simulink model "NMC_batt_model_100_1dot5C"  (R2023b)
settings: Solver=FixedStepAuto  StartTime=0.0  StopTime=10^7  FixedStep=50
undefined symbols (not defined in the file or in its folder): DiscIntNeverNeededParam, sigbuilder_block
libraries: batteryecm_lib x100, fl_lib x15, nesl_utility x10, simulink x2, dspswit3 x2
(part 1 of 4)
settings Model: Creator=OADEBAJO  LastModifiedBy=OADEBAJO
settings SolverCC: ZeroCrossAlgorithm=Adaptive

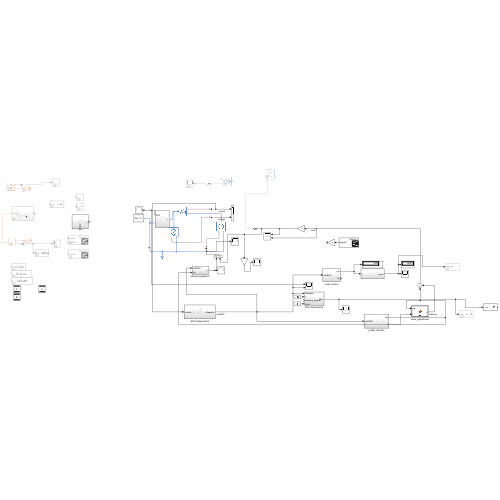
[thumbnail: Simulink's stored preview of the top-level diagram]
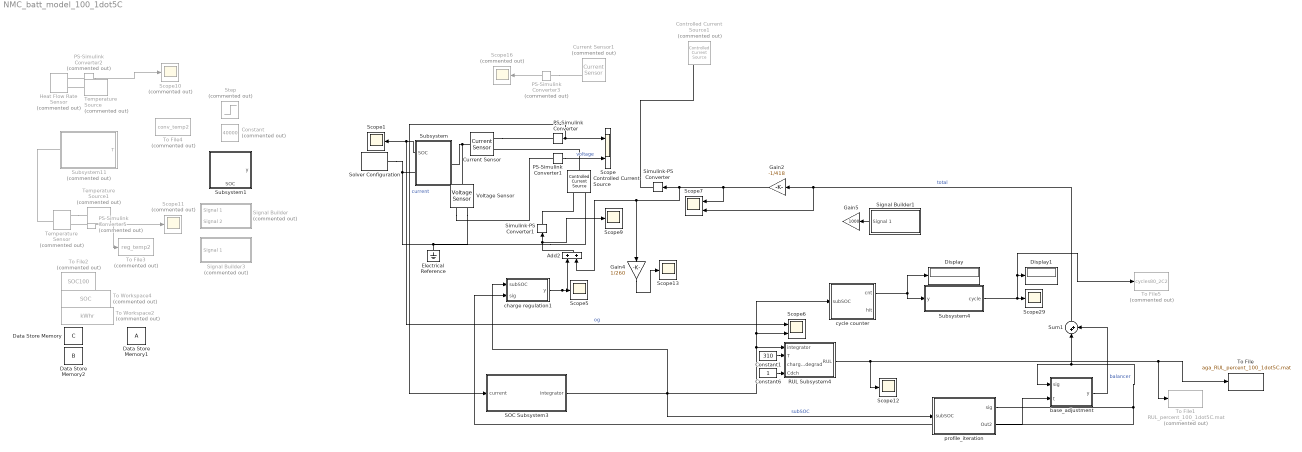
== system NMC_batt_model_100_1dot5C ==
  Add2 : Sum
  Constant : Constant  Commented=on  Value=40000
  Constant1 : Constant  Value=310
  Constant6 : Constant
  Controlled Current Source : fl_lib/Electrical/Electrical Sources/Controlled Current Source
  Controlled Current Source1 : fl_lib/Electrical/Electrical Sources/Controlled Current Source  Commented=on
  Current Sensor : fl_lib/Electrical/Electrical Sensors/Current Sensor
  Current Sensor1 : fl_lib/Electrical/Electrical Sensors/Current Sensor  Commented=on
  Data Store Memory : DataStoreMemory  DataStoreName=C  ReadBeforeWriteMsg=warning  WriteAfterWriteMsg=warning  WriteAfterReadMsg=warning  InitialValue=|  ShowAdditionalParam=off  OutDataTypeStr=double
      | [2000
      | 31300
      | 31300
      | 31300
      | 31300
      | 31300
      | 31300
      | 31300
      | 31300
      | 31300
      | 31300
      | 31300
      | 31300
      | 31300
      | 31300
      | 31300
      | 31300
      | 31300
      | 31300
      | 31300
      | 31300
      | 31300
      | 30655
      | 29990.5
      | 29960.5
      | 32605
      | 35210
      | 34000
      | 30450
      | 30526.67
      | 30460
      | 32000
      | 31716.67
      | 39932.84
      | 39885.07
      | 39837.31
      | 39789.55
      | 39212.64
      | 39210.82
      | 39209
      | 39207.18
      | 39205.36
      | 39203.55
      | 39201.73
      | 39199.91
      | 39198.09
      | 39196.27
      | 39194.45
      | 39192.64
      | 39190.82
      | 39189
      | 39187.18
      | 39185.36
      | 39183.55
      | 39181.73
      | 39179.91
      | 39178.09
      | 39176.27
      | 39174.45
      | 39024.33
      | 38949.38
      | 38948.69
      | 38948
      | 38947.31
      | 38946.62
      | 38945.93
      | 38945.24
      | 38944.55
      | 38943.86
      | 38943.17
      | 38942.48
      | 38941.79
      | 38941.1
      | 38940.41
      | 38939.72
      | 38939.03
      | 38938.34
      | 38937.65
      | 38936.96
      | 38936.27
      | 38935.58
      | 38934.89
      | 38934.2
      | 38933.51
      | 38932.82
      | 38932.13
      | 38931.44
      | 38930.75
      | 38930.06
      | 38929.37
      | 38928.68
      | 38927.99
      | 38927.3
      | 38926.61
      | 38925.92
      | 38925.23
      | 38924.54
      | 38923.85
      | 38923.16
      | 38922.47
      | 38921.79
      | 38921.1
      | 38920.41
      | 38919.72
      | 38919.03
      | 38918.34
      | 38917.65
      | 38916.96
      | 38916.27
      | 38915.58
      | 38914.89
      | 38914.2
      | 38913.51
      | 38912.82
      | 38912.13
      | 38911.44
      | 38910.75
      | 38910.06
      | 38909.37
      | 38908.68
      | 38907.99
      | 38907.3
      | 38906.61
      | 38905.92
      | 38905.23
      | 38904.54
      | 38903.85
      | 38903.16
      | 38902.47
      | 38901.78
      | 38901.09
      | 38900.4
      | 38899.71
      | 38899.02
      | 38898.33
      | 38897.64
      | 38896.95
      | 38896.26
      | 38895.57
      | 38894.88
      | 38894.19
      | 38893.5
      | 38892.81
      | 38892.12
      | 38891.43
      | 38890.74
      | 38890.05
      | 38889.36
      | 38888.67
      | 38887.98
      | 38887.29
      | 38886.6
      | 38885.91
      | 38885.22
      | 38884.53
      | 38883.84
      | 38883.15
      | 38882.46
      | 38881.77
      | 38881.08
      | 38880.39
      | 38879.7
      | 38879.01
      | 38878.32
      | 38877.63
      | 38876.94
      | 38876.25
      | 38875.56
      | 38874.87
      | 38874.19
      | 38873.5
      | 38872.81
      | 38872.12
      | 38871.43
      | 38870.74
      | 38870.05
      | 38869.36
      | 38868.67
      | 38867.98
      | 38867.29
      | 38866.6
      | 38865.91
      | 38865.22
      | 38864.53
      | 38863.84
      | 38863.15
      | 38862.46
      | 38861.77
      | 38861.08
      | 38860.39
      | 38859.7
      | 38859.01
      | 38858.32
      | 38857.63
      | 38856.94
      | 38856.25
      | 38855.56
      | 38854.87
      | 38854.18
      | 38853.49
      | 38852.8
      | 38852.11
      | 38851.42
      | 38850.73
      | 38850.04
      | 38849.35
      | 38848.66
      | 38847.97
      | 38847.28
      | 38846.59
      | 38845.9
      | 38845.21
      | 38844.52
      | 38843.83
      | 38843.14
      | 38842.45
      | 38841.76
      | 38841.07
      | 38840.38
      | 38839.69
      | 38839
      | 38838.31
      | 38837.62
      | 38836.93
      | 38836.24
      | 38835.55
      | 38834.86
      | 38834.17
      | 38833.48
      | 38832.79
      | 38832.1
      | 38831.41
      | 38830.72
      | 38830.03
      | 36768.41
      | 35227.5
      | 34141.5
      | 35942.5
      | 33093.33
      | 29998.33
      | 29290
      | 29290
      | 32756.67
      | 30673.33
      | 30960
      | 30067.5
      | 30017.5
      | 2000]
  Data Store Memory1 : DataStoreMemory  ReadBeforeWriteMsg=warning  WriteAfterWriteMsg=warning  WriteAfterReadMsg=warning  InitialValue=|  ShowAdditionalParam=off  OutDataTypeStr=double
      | [2000
      | 31300
      | 31300
      | 31300
      | 31300
      | 31300
      | 31300
      | 31300
      | 31300
      | 30005.5
      | 32605
      | 30040
      | 30460
      | 37653
      | 39837.31343
      | 39211.72727
      | 39207.18182
      | 39202.63636
      | 39198.09091
      | 39193.54545
      | 39189
      | 39184.45455
      | 39179.90909
      | 39175.36364
      | 38949.37913
      | 38947.6545
      | 38945.92986
      | 38944.20523
      | 38942.4806
      | 38940.75596
      | 38939.03133
      | 38937.3067
      | 38935.58206
      | 38933.85743
      | 38932.1328
      | 38930.40816
      | 38928.68353
      | 38926.9589
      | 38925.23426
      | 38923.50963
      | 38921.785
      | 38920.06036
      | 38918.33573
      | 38916.6111
      | 38914.88646
      | 38913.16183
      | 38911.43719
      | 38909.71256
      | 38907.98793
      | 38906.26329
      | 38904.53866
      | 38902.81403
      | 38901.08939
      | 38899.36476
      | 38897.64013
      | 38895.91549
      | 38894.19086
      | 38892.46623
      | 38890.74159
      | 38889.01696
      | 38887.29233
      | 38885.56769
      | 38883.84306
      | 38882.11842
      | 38880.39379
      | 38878.66916
      | 38876.94452
      | 38875.21989
      | 38873.49526
      | 38871.77062
      | 38870.04599
      | 38868.32136
      | 38866.59672
      | 38864.87209
      | 38863.14746
      | 38861.42282
      | 38859.69819
      | 38857.97356
      | 38856.24892
      | 38854.52429
      | 38852.79966
      | 38851.07502
      | 38849.35039
      | 38847.62575
      | 38845.90112
      | 38844.17649
      | 38842.45185
      | 38840.72722
      | 38839.00259
      | 38837.27795
      | 38835.55332
      | 38833.82869
      | 38832.10405
      | 38830.37942
      | 35227.5
      | 36585
      | 29290
      | 32820
      | 16000
      | 2000]
  Data Store Memory2 : DataStoreMemory  DataStoreName=B  WriteAfterWriteMsg=warning  InitialValue=|  ShowAdditionalParam=off  OutDataTypeStr=double
      | [2000
      | 15000
      | 30000
      | 30004.2016806723
      | 30008.4033613445
      | 30012.6050420168
      | 30016.8067226891
      | 30021.0084033613
      | 30025.2100840336
      | 30029.4117647059
      | 30033.6134453782
      | 30037.8151260504
      | 30042.0168067227
      | 30046.2184873950
      | 30050.4201680672
      | 30054.6218487395
      | 30058.8235294118
      | 30063.0252100840
      | 30067.2268907563
      | 30071.4285714286
      | 30075.6302521008
      | 30079.8319327731
      | 30084.0336134454
      | 30088.2352941176
      | 30092.4369747899
      | 30096.6386554622
      | 30100.8403361345
      | 30105.0420168067
      | 30109.2436974790
      | 30113.4453781513
      | 30117.6470588235
      | 30121.8487394958
      | 30126.0504201681
      | 30130.2521008403
      | 30134.4537815126
      | 30138.6554621849
      | 30142.8571428571
      | 30147.0588235294
      | 30151.2605042017
      | 30155.4621848739
      | 30159.6638655462
      | 30163.8655462185
      | 30168.0672268908
      | 30172.2689075630
      | 30176.4705882353
      | 30180.6722689076
      | 30184.8739495798
      | 30189.0756302521
      | 30193.2773109244
      | 30197.4789915966
      | 30201.6806722689
      | 30205.8823529412
      | 30210.0840336134
      | 30214.2857142857
      | 30218.4873949580
      | 30222.6890756303
      | 30226.8907563025
      | 30231.0924369748
      | 30235.2941176471
      | 30239.4957983193
      | 30243.6974789916
      | 30247.8991596639
      | 30252.1008403361
      | 30256.3025210084
      | 30260.5042016807
      | 30264.7058823529
      | 30268.9075630252
      | 30273.1092436975
      | 30277.3109243698
      | 30281.5126050420
      | 30285.7142857143
      | 30289.9159663866
      | 30294.1176470588
      | 30298.3193277311
      | 30302.5210084034
      | 30306.7226890756
      | 30310.9243697479
      | 30315.1260504202
      | 30319.3277310924
      | 30323.5294117647
      | 30327.7310924370
      | 30331.9327731092
      | 30336.1344537815
      | 30340.3361344538
      | 30344.5378151261
      | 30348.7394957983
      | 30352.9411764706
      | 30357.1428571429
      | 30361.3445378151
      | 30365.5462184874
      | 30369.7478991597
      | 30373.9495798319
      | 30378.1512605042
      | 30382.3529411765
      | 30386.5546218487
      | 30390.7563025210
      | 30394.9579831933
      | 30399.1596638655
      | 30403.3613445378
      | 30407.5630252101
      | 30411.7647058824
      | 30415.9663865546
      | 30420.1680672269
      | 30424.3697478992
      | 30428.5714285714
      | 30432.7731092437
      | 30436.9747899160
      | 30441.1764705882
      | 30445.3781512605
      | 30449.5798319328
      | 30453.7815126050
      | 30457.9831932773
      | 30462.1848739496
      | 30466.3865546218
      | 30470.5882352941
      | 30474.7899159664
      | 30478.9915966387
      | 30483.1932773109
      | 30487.3949579832
      | 30491.5966386555
      | 30495.7983193277
      | 30500
      | 30504.2016806723
      | 30508.4033613445
      | 30512.6050420168
      | 30516.8067226891
      | 30521.0084033613
      | 30525.2100840336
      | 30529.4117647059
      | 30533.6134453782
      | 30537.8151260504
      | 30542.0168067227
      | 30546.2184873950
      | 30550.4201680672
      | 30554.6218487395
      | 30558.8235294118
      | 30563.0252100840
      | 30567.2268907563
      | 30571.4285714286
      | 30575.6302521008
      | 30579.8319327731
      | 30584.0336134454
      | 30588.2352941176
      | 30592.4369747899
      | 30596.6386554622
      | 30600.8403361345
      | 30605.0420168067
      | 30609.2436974790
      | 30613.4453781513
      | 30617.6470588235
      | 30621.8487394958
      | 30626.0504201681
      | 30630.2521008403
      | 30634.4537815126
      | 30638.6554621849
      | 30642.8571428571
      | 30647.0588235294
      | 30651.2605042017
      | 30655.4621848739
      | 30659.6638655462
      | 30663.8655462185
      | 30668.0672268908
      | 30672.2689075630
      | 30676.4705882353
      | 30680.6722689076
      | 30684.8739495798
      | 30689.0756302521
      | 30693.2773109244
      | 30697.4789915966
      | 30701.6806722689
      | 30705.8823529412
      | 30710.0840336134
      | 30714.2857142857
      | 30718.4873949580
      | 30722.6890756303
      | 30726.8907563025
      | 30731.0924369748
      | 30735.2941176471
      | 30739.4957983193
      | 30743.6974789916
      | 30747.8991596639
      | 30752.1008403361
      | 30756.3025210084
      | 30760.5042016807
      | 30764.7058823529
      | 30768.9075630252
      | 30773.1092436975
      | 30777.3109243698
      | 30781.5126050420
      | 30785.7142857143
      | 30789.9159663866
      | 30794.1176470588
      | 30798.3193277311
      | 30802.5210084034
      | 30806.7226890756
      | 30810.9243697479
      | 30815.1260504202
      | 30819.3277310924
      | 30823.5294117647
      | 30827.7310924370
      | 30831.9327731092
      | 30836.1344537815
      | 30840.3361344538
      | 30844.5378151261
      | 30848.7394957983
      | 30852.9411764706
      | 30857.1428571429
      | 30861.3445378151
      | 30865.5462184874
      | 30869.7478991597
      | 30873.9495798319
      | 30878.1512605042
      | 30882.3529411765
      | 30886.5546218487
      | 30890.7563025210
      | 30894.9579831933
      | 30899.1596638655
      | 30903.3613445378
      | 30907.5630252101
      | 30911.7647058824
      | 30915.9663865546
      | 30920.1680672269
      | 30924.3697478992
      | 30928.5714285714
      | 30932.7731092437
      | 30936.9747899160
      | 30941.1764705882
      | 30945.3781512605
      | 30949.5798319328
      | 30953.7815126050
      | 30957.9831932773
      | 30962.1848739496
      | 30966.3865546218
      | 30970.5882352941
      | 30974.7899159664
      | 30978.9915966387
      | 30983.1932773109
      | 30987.3949579832
      | 30991.5966386555
      | 30995.7983193277
      | 40000
      | 40000
      | 40000
      | 40000
      | 40000
      | 40000
      | 40000
      | 40000
      | 40000
      | 40000
      | 40000
      | 40000
      | 40000
      | 40000
      | 40000
      | 40000
      | 40000
      | 40000
      | 40000
      | 40000
      | 40000
      | 40000
      | 40000
      | 40000
      | 40000
      | 40000
      | 40000
      | 40000
      | 40000
      | 40000
      | 40000
      | 40000
      | 40000
      | 40000
      | 40000
      | 40000
      | 40000
      | 40000
      | 40000
      | 40000
      | 40000
      | 40000
      | 40000
      | 40000
      | 40000
      | 40000
      | 40000
      | 40000
      | 40000
      | 40000
      | 40000
      | 40000
      | 40000
      | 40000
      | 40000
      | 40000
      | 40000
      | 40000
      | 40000
      | 40000
      | 40000
      | 40000
      | 40000
      | 40000
      | 40000
      | 40000
      | 40000
      | 40000
      | 40000
      | 40000
      | 40000
      | 40000
      | 40000
      | 40000
      | 40000
      | 40000
      | 40000
      | 40000
      | 40000
      | 40000
      | 40000
      | 40000
      | 40000
      | 40000
      | 40000
      | 40000
      | 40000
      | 40000
      | 40000
      | 40000
      | 40000
      | 40000
      | 40000
      | 40000
      | 40000
      | 40000
      | 40000
      | 40000
      | 40000
      | 40000
      | 40000
      | 40000
      | 40000
      | 40000
      | 40000
      | 40000
      | 40000
      | 40000
      | 40000
      | 40000
      | 40000
      | 40000
      | 40000
      | 40000
      | 40000
      | 40000
      | 40000
      | 40000
      | 40000
      | 40000
      | 40000
      | 40000
      | 40000
      | 40000
      | 40000
      | 40000
      | 40000
      | 40000
      | 40000
      | 40000
      | 40000
      | 40000
      | 40000
      | 40000
      | 40000
      | 40000
      | 40000
      | 40000
      | 40000
      | 40000
      | 40000
      | 40000
      | 40000
      | 40000
      | 40000
      | 40000
      | 40000
      | 40000
      | 40000
      | 40000
      | 40000
      | 40000
      | 40000
      | 40000
      | 40000
      | 40000
      | 40000
      | 40000
      | 40000
      | 40000
      | 38000
      | 38000
      | 38000
      | 38000
      | 38000
      | 38000
      | 38000
      | 38000
      | 38000
      | 38000
      | 38000
      | 38000
      | 38000
      | 38000
      | 38000
      | 38000
      | 38000
      | 38000
      | 38000
      | 38000
      | 38000
      | 38000
      | 38000
      | 38000
      | 38000
      | 38000
      | 38000
      | 38000
      | 38000
      | 38000
      | 38000
      | 38000
      | 38000
      | 38000
      | 38000
      | 38000
      | 38000
      | 38000
      | 38000
      | 38000
      | 38000
      | 38000
      | 38000
      | 38000
      | 38000
      | 38000
      | 38000
      | 38000
      | 38000
      | 38000
      | 38000
      | 38000
      | 38000
      | 38000
      | 38000
      | 38000
      | 38000
      | 38000
      | 38000
      | 38000
      | 38000
      | 38000
      | 38000
      | 38000
      | 38000
      | 38000
      | 38000
      | 38000
      | 38000
      | 38000
      | 38000
      | 38000
      | 38000
      | 38000
      | 38000
      | 38000
      | 38000
      | 38000
      | 38000
      | 38000
      | 38000
      | 38000
      | 38000
      | 38000
      | 38000
      | 38000
      | 38000
      | 38000
      | 38000
      | 38000
      | 38000
      | 38000
      | 38000
      | 38000
      | 38000
      | 38000
      | 38000
      | 38000
      | 38000
      | 38000
      | 38000
      | 38000
      | 38000
      | 38000
      | 38000
      | 38000
      | 38000
      | 38000
      | 38000
      | 38000
      | 38000
      | 38000
      | 38000
      | 38000
      | 38000
      | 38000
      | 38000
      | 38000
      | 38000
      | 38000
      | 38000
      | 38000
      | 38000
      | 38000
      | 38000
      | 38000
      | 38000
      | 38000
      | 38000
      | 38000
      | 38000
      | 38000
      | 38000
      | 38000
      | 38000
      | 38000
      | 38000
      | 38000
      | 38000
      | 38000
      | 38000
      | 38000
      | 38000
      | 38000
      | 38000
      | 38000
      | 38000
      | 38000
      | 38000
      | 38000
      | 36000
      | 36000
      | 36000
      | 36000
      | 36000
      | 36000
      | 36000
      | 36000
      | 36000
      | 36000
      | 36000
      | 36000
      | 36000
      | 36000
      | 36000
      | 36000
      | 36000
      | 36000
      | 36000
      | 36000
      | 36000
      | 36000
      | 36000
      | 36000
      | 36000
      | 36000
      | 36000
      | 36000
      | 36000
      | 36000
      | 36000
      | 36000
      | 36000
      | 36000
      | 36000
      | 36000
      | 36000
      | 36000
      | 36000
      | 36000
      | 36000
      | 36000
      | 36000
      | 36000
      | 36000
      | 36000
      | 36000
      | 36000
      | 36000
      | 36000
      | 36000
      | 36000
      | 36000
      | 36000
      | 36000
      | 36000
      | 36000
      | 36000
      | 36000
      | 36000
      | 36000
      | 36000
      | 36000
      | 36000
      | 36000
      | 36000
      | 36000
      | 36000
      | 36000
      | 36000
      | 36000
      | 36000
      | 36000
      | 36000
      | 36000
      | 36000
      | 36000
      | 36000
      | 36000
      | 36000
      | 36000
      | 36000
      | 36000
      | 36000
      | 36000
      | 36000
      | 36000
      | 36000
      | 36000
      | 36000
      | 36000
      | 36000
      | 36000
      | 36000
      | 36000
      | 36000
      | 36000
      | 36000
      | 36000
      | 36000
      | 36000
      | 36000
      | 36000
      | 36000
      | 36000
      | 36000
      | 36000
      | 36000
      | 36000
      | 36000
      | 36000
      | 36000
      | 36000
      | 36000
      | 36000
      | 36000
      | 36000
      | 36000
      | 36000
      | 36000
      | 36000
      | 36000
      | 36000
      | 36000
      | 36000
      | 36000
      | 36000
      | 36000
      | 36000
      | 36000
      | 36000
      | 36000
      | 36000
      | 36000
      | 36000
      | 36000
      | 36000
      | 36000
      | 36000
      | 36000
      | 36000
      | 36000
      | 36000
      | 36000
      | 36000
      | 36000
      | 36000
      | 36000
      | 36000
      | 36000
      | 36000
      | 36000
      | 36000
      | 36000
      | 36000
      | 36000
      | 36000
      | 36000
      | 36000
      | 36000
      | 36000
      | 36000
      | 36000
      | 36000
      | 36000
      | 36000
      | 36000
      | 36000
      | 36000
      | 36000
      | 36000
      | 36000
      | 36000
      | 36000
      | 36000
      | 36000
      | 36000
      | 36000
      | 36000
      | 36000
      | 36000
      | 36000
      | 36000
      | 36000
      | 36000
      | 36000
      | 36000
      | 36000
      | 36000
      | 36000
      | 36000
      | 36000
      | 36000
      | 36000
      | 36000
      | 36000
      | 36000
      | 36000
      | 36000
      | 36000
      | 36000
      | 36000
      | 36000
      | 36000
      | 36000
      | 36000
      | 36000
      | 36000
      | 36000
      | 36000
      | 36000
      | 36000
      | 36000
      | 36000
      | 36000
      | 36000
      | 36000
      | 36000
      | 36000
      | 36000
      | 36000
      | 36000
      | 36000
      | 36000
      | 36000
      | 36000
      | 36000
      | 36000
      | 36000
      | 36000
      | 36000
      | 36000
      | 36000
      | 36000
      | 36000
      | 36000
      | 36000
      | 36000
      | 36000
      | 36000
      | 36000
      | 36000
      | 36000
      | 36000
      | 36000
      | 36000
      | 36000
      | 36000
      | 36000
      | 36000
      | 36000
      | 36000
      | 36000
      | 36000
      | 36000
      | 36000
      | 36000
      | 36000
      | 36000
      | 36000
      | 36000
      | 36000
      | 36000
      | 36000
      | 36000
      | 36000
      | 36000
      | 36000
      | 36000
      | 36000
      | 36000
      | 36000
      | 36000
      | 36000
      | 36000
      | 36000
      | 36000
      | 36000
      | 36000
      | 36000
      | 36000
      | 36000
      | 36000
      | 36000
      | 36000
      | 36000
      | 36000
      | 36000
      | 36000
      | 36000
      | 36000
      | 36000
      | 36000
      | 36000
      | 36000
      | 36000
      | 36000
      | 36000
      | 36000
      | 36000
      | 36000
      | 36000
      | 36000
      | 36000
      | 36000
      | 36000
      | 36000
      | 36000
      | 36000
      | 36000
      | 36000
      | 36000
      | 36000
      | 36000
      | 36000
      | 36000
      | 36000
      | 36000
      | 36000
      | 36000
      | 36000
      | 36000
      | 36000
      | 36000
      | 36000
      | 36000
      | 36000
      | 36000
      | 36000
      | 36000
      | 36000
      | 36000
      | 36000
      | 36000
      | 36000
      | 36000
      | 36000
      | 36000
      | 36000
      | 36000
      | 36000
      | 36000
      | 36000
      | 36000
      | 36000
      | 36000
      | 36000
      | 36000
      | 36000
      | 36000
      | 36000
      | 36000
      | 36000
      | 36000
      | 36000
      | 36000
      | 36000
      | 36000
      | 36000
      | 36000
      | 36000
      | 36000
      | 36000
      | 36000
      | 36000
      | 36000
      | 36000
      | 36000
      | 36000
      | 36000
      | 36000
      | 36000
      | 36000
      | 36000
      | 36000
      | 36000
      | 36000
      | 36000
      | 36000
      | 36000
      | 36000
      | 36000
      | 36000
      | 36000
      | 36000
      | 36000
      | 36000
      | 36000
      | 36000
      | 36000
      | 36000
      | 36000
      | 36000
      | 36000
      | 36000
      | 36000
      | 36000
      | 36000
      | 36000
      | 36000
      | 36000
      | 36000
      | 36000
      | 36000
      | 36000
      | 36000
      | 36000
      | 36000
      | 36000
      | 36000
      | 36000
      | 36000
      | 36000
      | 36000
      | 36000
      | 36000
      | 36000
      | 36000
      | 36000
      | 36000
      | 36000
      | 36000
      | 36000
      | 36000
      | 36000
      | 36000
      | 36000
      | 36000
      | 36000
      | 36000
      | 36000
      | 36000
      | 36000
      | 36000
      | 36000
      | 36000
      | 36000
      | 36000
      | 36000
      | 36000
      | 36000
      | 36000
      | 36000
      | 36000
      | 36000
      | 36000
      | 36000
      | 36000
      | 36000
      | 36000
      | 36000
      | 36000
      | 36000
      | 36000
      | 36000
      | 36000
      | 36000
      | 36000
      | 36000
      | 36000
      | 36000
      | 36000
      | 36000
      | 36000
      | 36000
      | 36000
      | 36000
      | 36000
      | 36000
      | 36000
      | 36000
      | 36000
      | 36000
      | 36000
      | 36000
      | 36000
      | 36000
      | 36000
      | 36000
      | 36000
      | 36000
      | 36000
      | 36000
      | 36000
      | 36000
      | 36000
      | 36000
      | 36000
      | 36000
      | 36000
      | 36000
      | 36000
      | 36000
      | 36000
      | 36000
      | 36000
      | 36000
      | 36000
      | 36000
      | 36000
      | 36000
      | 36000
      | 36000
      | 36000
      | 36000
      | 36000
      | 36000
      | 36000
      | 36000
      | 36000
      | 36000
      | 36000
      | 36000
      | 36000
      | 36000
      | 36000
      | 36000
      | 36000
      | 36000
      | 36000
      | 36000
      | 36000
      | 36000
      | 36000
      | 36000
      | 36000
      | 36000
      | 36000
      | 36000
      | 36000
      | 36000
      | 36000
      | 36000
      | 36000
      | 36000
      | 36000
      | 36000
      | 36000
      | 36000
      | 36000
      | 36000
      | 36000
      | 36000
      | 36000
      | 36000
      | 36000
      | 36000
      | 36000
      | 36000
      | 36000
      | 36000
      | 36000
      | 36000
      | 36000
      | 36000
      | 36000
      | 36000
      | 36000
      | 36000
      | 36000
      | 36000
      | 36000
      | 36000
      | 36000
      | 36000
      | 36000
      | 36000
      | 36000
      | 36000
      | 36000
      | 36000
      | 36000
      | 36000
      | 36000
      | 36000
      | 36000
      | 36000
      | 36000
      | 36000
      | 36000
      | 36000
      | 36000
      | 36000
      | 36000
      | 36000
      | 36000
      | 36000
      | 36000
      | 36000
      | 36000
      | 36000
      | 36000
      | 36000
      | 36000
      | 36000
      | 36000
      | 36000
      | 36000
      | 36000
      | 36000
      | 36000
      | 36000
      | 36000
      | 36000
      | 36000
      | 36000
      | 36000
      | 36000
      | 36000
      | 36000
      | 36000
      | 36000
      | 36000
      | 36000
      | 36000
      | 36000
      | 36000
      | 36000
      | 36000
      | 36000
      | 36000
      | 36000
      | 36000
      | 36000
      | 36000
      | 36000
      | 36000
      | 36000
      | 36000
      | 36000
      | 36000
      | 36000
      | 36000
      | 36000
      | 36000
      | 36000
      | 36000
      | 36000
      | 36000
      | 36000
      | 36000
      | 36000
      | 36000
      | 36000
      | 36000
      | 36000
      | 36000
      | 36000
      | 36000
      | 36000
      | 36000
      | 36000
      | 36000
      | 36000
      | 36000
      | 36000
      | 36000
      | 36000
      | 36000
      | 36000
      | 36000
      | 36000
      | 36000
      | 36000
      | 36000
      | 36000
      | 36000
      | 36000
      | 36000
      | 36000
      | 36000
      | 36000
      | 36000
      | 36000
      | 36000
      | 36000
      | 36000
      | 36000
      | 36000
      | 36000
      | 36000
      | 36000
      | 36000
      | 36000
      | 36000
      | 36000
      | 36000
      | 36000
      | 36000
      | 36000
      | 36000
      | 36000
      | 36000
      | 36000
      | 36000
      | 36000
      | 36000
      | 36000
      | 36000
      | 36000
      | 36000
      | 36000
      | 36000
      | 36000
      | 36000
      | 36000
      | 36000
      | 36000
      | 36000
      | 36000
      | 36000
      | 36000
      | 36000
      | 36000
      | 36000
      | 36000
      | 36000
      | 36000
      | 36000
      | 36000
      | 36000
      | 36000
      | 36000
      | 36000
      | 36000
      | 36000
      | 36000
      | 36000
      | 36000
      | 36000
      | 36000
      | 36000
      | 36000
      | 36000
      | 36000
      | 36000
      | 36000
      | 36000
      | 36000
      | 36000
      | 36000
      | 36000
      | 36000
      | 36000
      | 36000
      | 36000
      | 36000
      | 36000
      | 36000
      | 36000
      | 36000
      | 36000
      | 36000
      | 36000
      | 36000
      | 36000
      | 36000
      | 36000
      | 36000
      | 36000
      | 36000
      | 36000
      | 36000
      | 36000
      | 36000
      | 36000
      | 36000
      | 36000
      | 36000
      | 36000
      | 36000
      | 36000
      | 36000
      | 36000
      | 36000
      | 36000
      | 36000
      | 36000
      | 36000
      | 36000
      | 36000
      | 36000
      | 36000
      | 36000
      | 36000
      | 36000
      | 36000
      | 36000
      | 36000
      | 36000
      | 36000
      | 36000
      | 36000
      | 36000
      | 36000
      | 36000
      | 36000
      | 36000
      | 36000
      | 36000
      | 36000
      | 36000
      | 36000
      | 36000
      | 36000
      | 36000
      | 36000
      | 36000
      | 36000
      | 36000
      | 36000
      | 36000
      | 36000
      | 36000
      | 36000
      | 36000
      | 36000
      | 36000
      | 36000
      | 36000
      | 36000
      | 36000
      | 36000
      | 36000
      | 36000
      | 36000
      | 36000
      | 36000
      | 36000
      | 36000
      | 36000
      | 36000
      | 36000
      | 36000
      | 36000
      | 36000
      | 36000
      | 36000
      | 36000
      | 36000
      | 36000
      | 36000
      | 36000
      | 36000
      | 36000
      | 36000
      | 36000
      | 36000
      | 36000
      | 36000
      | 36000
      | 36000
      | 36000
      | 36000
      | 36000
      | 36000
      | 36000
      | 36000
      | 36000
      | 36000
      | 36000
      | 36000
      | 36000
      | 36000
      | 36000
      | 36000
      | 36000
      | 36000
      | 36000
      | 36000
      | 36000
      | 36000
      | 36000
      | 36000
      | 36000
      | 36000
      | 36000
      | 36000
      | 36000
      | 36000
      | 36000
      | 36000
      | 36000
      | 36000
      | 36000
      | 36000
      | 36000
      | 36000
      | 36000
      | 36000
      | 36000
      | 36000
      | 36000
      | 36000
      | 36000
      | 36000
      | 36000
      | 36000
      | 36000
      | 36000
      | 36000
      | 36000
      | 36000
      | 36000
      | 36000
      | 36000
      | 36000
      | 36000
      | 36000
      | 36000
      | 36000
      | 36000
      | 36000
      | 36000
      | 36000
      | 36000
      | 36000
      | 36000
      | 36000
      | 36000
      | 36000
      | 36000
      | 36000
      | 36000
      | 36000
      | 36000
      | 36000
      | 36000
      | 36000
      | 36000
      | 36000
      | 36000
      | 36000
      | 36000
      | 36000
      | 36000
      | 36000
      | 36000
      | 36000
      | 36000
      | 36000
      | 36000
      | 36000
      | 36000
      | 36000
      | 36000
      | 36000
      | 36000
      | 36000
      | 36000
      | 36000
      | 36000
      | 36000
      | 36000
      | 36000
      | 36000
      | 36000
      | 36000
      | 36000
      | 36000
      | 36000
      | 36000
      | 36000
      | 36000
      | 36000
      | 36000
      | 36000
      | 36000
      | 36000
      | 36000
      | 36000
      | 36000
      | 36000
      | 36000
      | 36000
      | 36000
      | 36000
      | 36000
      | 36000
      | 36000
      | 36000
      | 36000
      | 36000
      | 36000
      | 36000
      | 36000
      | 36000
      | 36000
      | 36000
      | 36000
      | 36000
      | 36000
      | 36000
      | 36000
      | 36000
      | 36000
      | 36000
      | 36000
      | 36000
      | 36000
      | 36000
      | 36000
      | 36000
      | 36000
      | 36000
      | 36000
      | 36000
      | 36000
      | 36000
      | 36000
      | 36000
      | 36000
      | 36000
      | 36000
      | 36000
      | 36000
      | 36000
      | 36000
      | 36000
      | 36000
      | 36000
      | 36000
      | 36000
      | 36000
      | 36000
      | 36000
      | 36000
      | 36000
      | 36000
      | 36000
      | 36000
      | 36000
      | 36000
      | 36000
      | 36000
      | 36000
      | 36000
      | 36000
      | 36000
      | 36000
      | 36000
      | 36000
      | 36000
      | 36000
      | 36000
      | 36000
      | 36000
      | 36000
      | 36000
      | 36000
      | 36000
      | 35850.0000000000
      | 35700.0000000000
      | 35550
      | 35400
      | 35250
      | 35100
      | 34950
      | 34800
      | 34650
      | 34500
      | 34350
      | 34200
      | 34050
      | 33900
      | 33750
      | 33600
      | 33450
      | 33300
      | 33150
      | 33000
      | 33000
      | 33000
      | 33000
      | 33000
      | 33000
      | 33000
      | 33000
      | 33000
      | 33000
      | 33000
      | 33000
      | 33000
      | 33000
      | 33000
      | 33000
      | 33000
      | 33000
      | 33000
      | 33000
      | 33000
      | 33000
      | 33000
      | 33000
      | 33000
      | 33000
      | 33000
      | 33000
      | 33000
      | 33000
      | 32000
      | 32000
      | 32000
      | 32000
      | 32000
      | 32000
      | 32000
      | 32000
      | 32000
      | 32000
      | 32000
      | 32000
      | 32000
      | 32000
      | 32000
      | 32000
      | 32000
      | 32000
      | 32000
      | 32000
      | 32000
      | 32000
      | 32000
      | 32000
      | 32000
      | 32000
      | 32000
      | 32000
      | 32000
      | 32000
      | 32000
      | 32000
      | 32000
      | 32000
      | 32000
      | 32000
      | 32000
      | 32000
      | 32000
      | 32000
      | 32000
      | 32000
      | 32000
      | 32000
      | 32000
      | 32000
      | 32000
      | 32000
      | 32000
      | 32000
      | 32000
      | 32000
      | 32000
      | 32000
      | 32000
      | 32000
      | 32000
      | 32000
      | 32000
      | 32000
      | 32000
      | 32000
      | 32000
      | 32000
      | 32000
      | 32000
      | 32000
      | 32000
      | 32000
      | 32000
      | 32000
      | 32000
      | 32000
      | 32000
      | 32000
      | 32000
      | 32000
      | 32000
      | 32000
      | 32000
      | 32000
      | 32000
      | 32000
      | 32000
      | 32000
      | 32000
      | 32000
      | 32000
      | 32000
      | 32000
      | 32000
      | 32000
      | 32000
      | 32000
      | 32000
      | 32000
      | 32000
      | 32000
      | 32000
      | 32000
      | 32000
      | 32000
      | 32000
      | 32000
      | 32000
      | 32000
      | 32000
      | 32000
      | 32000
      | 32000
      | 32000
      | 32000
      | 32000
      | 32000
      | 32000
      | 32000
      | 32000
      | 32000
      | 32000
      | 32000
      | 32000
      | 32000
      | 32000
      | 32000
      | 32000
      | 32000
      | 32000
      | 32000
      | 32000
      | 32000
      | 32000
      | 32000
      | 32000
      | 32000
      | 32000
      | 32000
      | 32000
      | 32000
      | 32000
      | 32000
      | 32000
      | 32000
      | 32000
      | 32000
      | 32000
      | 32000
      | 32000
      | 32000
      | 32000
      | 16000
      | 2000]
  Display : Display
  Display1 : Display
  Electrical Reference : fl_lib/Electrical/Electrical Elements/Electrical Reference
  Gain2 : Gain  Gain=-1/418
  Gain4 : Gain  Gain=1/260
  Gain5 : Gain  Gain=1000
  Heat Flow Rate Sensor : fl_lib/Thermal/Thermal Sensors/Heat Flow Rate Sensor  Commented=on
  PS-Simulink Converter : nesl_utility/PS-Simulink Converter  PhysicalDomain=network_engine_domain  SubClassName=ps_output  LeftPortType=input  RightPortType=output  PseudoPeriodic=off  Frequencies=[]  VectorFormat=inherit  Unit=inherit  AffineConversion=off
  PS-Simulink Converter1 : nesl_utility/PS-Simulink Converter  PhysicalDomain=network_engine_domain  SubClassName=ps_output  LeftPortType=input  RightPortType=output  PseudoPeriodic=off  Frequencies=[]  VectorFormat=inherit  Unit=inherit  AffineConversion=off
  PS-Simulink Converter2 : nesl_utility/PS-Simulink Converter  Commented=on  PhysicalDomain=network_engine_domain  SubClassName=ps_output  LeftPortType=input  RightPortType=output  PseudoPeriodic=off  Frequencies=[]  VectorFormat=inherit  Unit=inherit  AffineConversion=off
  PS-Simulink Converter3 : nesl_utility/PS-Simulink Converter  Commented=on  PhysicalDomain=network_engine_domain  SubClassName=ps_output  LeftPortType=input  RightPortType=output  PseudoPeriodic=off  Frequencies=[]  VectorFormat=inherit  Unit=inherit  AffineConversion=off
  PS-Simulink Converter5 : nesl_utility/PS-Simulink Converter  Commented=on  PhysicalDomain=network_engine_domain  SubClassName=ps_output  LeftPortType=input  RightPortType=output  PseudoPeriodic=off  Frequencies=[]  VectorFormat=inherit  Unit=inherit  AffineConversion=off
  RUL Subsystem4 : Subsystem
  SOC Subsystem3 : Subsystem
  Scope : Scope  NumInputPorts=2
  Scope{1,5,9,12..13,29} (6 alike) : Scope
  Scope10 : Scope  Commented=on
  Scope11 : Scope  Commented=on
  Scope16 : Scope  Commented=on
  Scope6 : Scope  NumInputPorts=2
  Scope7 : Scope  NumInputPorts=2
  Signal Builder : Subsystem  Tag=STV Subsys  Commented=on  LoadFcn=sigbuilder_block('load');  StartFcn=sigbuilder_block('start');  StopFcn=sigbuilder_block('stop');  ClipboardFcn=sigbuilder_block('clipboard');  mask(Sigbuilder block){tuvar=[0:10]}
      mask help: Simulink:masks:SigbuilderBlock_MD
      mask init:
      | if ~strcmp(get_param(bdroot(gcbh),'SimulationStatus'),'stopped') tuvar = sigbuilder_block('maskInit'); end
      settings: CopyFcn=sigbuilder_block('copy');  DeleteFcn=sigbuilder_block('delete');  ModelCloseFcn=sigbuilder_block('modelClose');  PreSaveFcn=sigbuilder_block('preSave');  PauseFcn=sigbuilder_block('pause');  ContinueFcn=sigbuilder_block('continue');  NameChangeFcn=sigbuilder_block('namechange');  OpenFcn=sigbuilder_block('open',[-104.25 -237 1428 771.75 ]);  CloseFcn=sigbuilder_block('close');
      mask Display: plot(0, 0, 100, 100,[2, 2, 32, 32, 2], [68, 8, 8, 68, 68],[32, 2], [38, 38], [32, 19, 2],[53, 60, 44], [32, 17, 17, 2],[16, 16, 31, 31]);txt = getActiveGroup(gcbh);text(2, 100, txt,'verticalAlignment', 'top');
  Signal Builder1 : Subsystem  Tag=STV Subsys  LoadFcn=sigbuilder_block('load');  StartFcn=sigbuilder_block('start');  StopFcn=sigbuilder_block('stop');  ClipboardFcn=sigbuilder_block('clipboard');  mask(Sigbuilder block){tuvar=[0:10]}
      mask help: Simulink:masks:SigbuilderBlock_MD
      mask init:
      | if ~strcmp(get_param(bdroot(gcbh),'SimulationStatus'),'stopped') tuvar = sigbuilder_block('maskInit'); end
      settings: CopyFcn=sigbuilder_block('copy');  DeleteFcn=sigbuilder_block('delete');  ModelCloseFcn=sigbuilder_block('modelClose');  PreSaveFcn=sigbuilder_block('preSave');  PauseFcn=sigbuilder_block('pause');  ContinueFcn=sigbuilder_block('continue');  NameChangeFcn=sigbuilder_block('namechange');  OpenFcn=sigbuilder_block('open',[6 -153 1428 641.25 ]);  CloseFcn=sigbuilder_block('close');
      mask Display: plot(0, 0, 100, 100,[2, 2, 32, 32, 2], [68, 8, 8, 68, 68],[32, 2], [38, 38], [32, 19, 2],[53, 60, 44], [32, 17, 17, 2],[16, 16, 31, 31]);txt = getActiveGroup(gcbh);text(2, 100, txt,'verticalAlignment', 'top');
  Signal Builder3 : Subsystem  Tag=STV Subsys  Commented=on  LoadFcn=sigbuilder_block('load');  StartFcn=sigbuilder_block('start');  StopFcn=sigbuilder_block('stop');  ClipboardFcn=sigbuilder_block('clipboard');  mask(Sigbuilder block){tuvar=[0:10]}
      mask help: Simulink:masks:SigbuilderBlock_MD
      mask init:
      | if ~strcmp(get_param(bdroot(gcbh),'SimulationStatus'),'stopped') tuvar = sigbuilder_block('maskInit'); end
      settings: CopyFcn=sigbuilder_block('copy');  DeleteFcn=sigbuilder_block('delete');  ModelCloseFcn=sigbuilder_block('modelClose');  PreSaveFcn=sigbuilder_block('preSave');  PauseFcn=sigbuilder_block('pause');  ContinueFcn=sigbuilder_block('continue');  NameChangeFcn=sigbuilder_block('namechange');  OpenFcn=sigbuilder_block('open',[6 30 1428 771.75 ]);  CloseFcn=sigbuilder_block('close');
      mask Display: plot(0, 0, 100, 100,[2, 2, 32, 32, 2], [68, 8, 8, 68, 68],[32, 2], [38, 38], [32, 19, 2],[53, 60, 44], [32, 17, 17, 2],[16, 16, 31, 31]);txt = getActiveGroup(gcbh);text(2, 100, txt,'verticalAlignment', 'top');
  Simulink-PS Converter : nesl_utility/Simulink-PS Converter  PhysicalDomain=network_engine_domain  SubClassName=ps_input  LeftPortType=input  RightPortType=output  PseudoPeriodic=off  Frequencies=[]  NoiseDistribution=none  NoiseParameters=[]  Unit=1  AffineConversion=off  FilteringAndDerivatives=provide  SimscapeFilterOrder=1  InputFilterTimeConstant=0.001  UdotUserProvided=0
  Simulink-PS Converter1 : nesl_utility/Simulink-PS Converter  PhysicalDomain=network_engine_domain  SubClassName=ps_input  LeftPortType=input  RightPortType=output  PseudoPeriodic=off  Frequencies=[]  NoiseDistribution=none  NoiseParameters=[]  Unit=1  AffineConversion=off  FilteringAndDerivatives=provide  SimscapeFilterOrder=1  InputFilterTimeConstant=0.001  UdotUserProvided=0
  Solver Configuration : nesl_utility/Solver Configuration  PhysicalDomain=network_engine_domain  SubClassName=solver  LeftPortType=input  RightPortType=generic  Tones=[]  Harmonics=[]  SimulateNoise=off  Profile=off  UseLocalSampling=off  EnableSwitchedLinearOptims=on  FrequencyDomain=off  UseCCode=off  RelTol=0.001  AbsTol=0.001  MinStep=1e-09  ToWorkspace=off  RevertToSquareIcSolve=off  NumHomotopyIterations=100  PhasorMode=off  PhasorModeNumHarmonics=1  ConsistencySolver=NEWTON_XTOL_AFTER_FTOL  IndexReductionMethod=DerivativeReplacement  DoDC=off  ResidualTolerance=1e-09  ConsistencyTolSource=GLOBAL  ConsistencyAbsTol=0.001  ConsistencyRelTol=0.001  ConsistencyTolFactor=1  UseLocalSolver=off  LocalSolverChoice=NE_BACKWARD_EULER_ADVANCER  ResolveIndetEquations=on  FunctionEvalNumThread=1  LocalSolverSampleTime=0.001  DoFixedCost=off  MaxNonlinIter=3  MaxModeIter=2  ComputeImpulses=off  ImpulseIterations=2  LinearAlgebra=auto  LinearAlgebraNumThread=0  EquationFormulation=NE_TIME_EF  DelaysMemoryBudget=1024  AutomaticFiltering=off  FilteringTimeConstant=0.001  PartitionStorageMethod=AS_NEEDED  PartitionMemoryBudget=1024  PartitionMethod=ROBUST  MultibodyUseLocalSolver=off  MultibodyLocalSolverChoice=ODE1  MultibodyLocalSolverSampleTime=0.001
  Step : Step  Commented=on  Time=5000  Before=40000  After=0  SampleTime=0
  Subsystem : Subsystem
  Subsystem1 : Subsystem
      settings: PortSchema="{\"entries\":[{\"content\":{\"sides\":[{\"content\":{},\"type\":\"ConnectorPlacement.EquallySpacedRectSide\",\"uuid\":\"dc57e3e7-2ad3-48c6-bee1-9177bcd0a010\"},{\"content\":{\"connectorIds\":[\"Out1\"],\"side\":\"RIGHT\"},\"type\":\"ConnectorPlacement.EquallySpacedRectSide\",\"uuid\":\"e6e1170d-dd5d-4d26-86f1-26d79cca7bfc\"},{\"content\":{\"side\":\"TOP\"},\"type\":\"ConnectorPlacement.EquallySpacedRectSide\",\"uuid\":\"c97b4621-c2d6-4890-b5f9-dcb0146c04f5\"},{\"content\":{\"connectorIds\":[\"In1\"],\"side\":\"BOTTOM\"},\"type\":\"ConnectorPlacement.EquallySpacedRectSide\",\"uuid\":\"d3809652-da81-49b5-8563-8bad0b471000\"}]},\"type\":\"ConnectorPlacement.EquallySpacedConnector\",\"uuid\":\"18947f02-c49d-41bd-b925-f09383c98f63\"}],\"packageUris\":[\"http://schema.mathworks.com/mf0/Connector/R2020b\"],\"version\":\"1.0\"}"
  Subsystem11 : Subsystem  Commented=on
  Subsystem4 : Subsystem
  Sum1 : Sum  Inputs=|++
  Temperature Sensor : fl_lib/Thermal/Thermal Sensors/Temperature Sensor  Commented=on  temperature_measure=foundation.enum.MeasurementReference.difference
  Temperature Source : fl_lib/Thermal/Thermal Sources/Temperature Source  Commented=on  temperature=293.15 K
  Temperature Source1 : fl_lib/Thermal/Thermal Sources/Temperature Source  Commented=on  temperature=293.15 K
  To File : ToFile  Filename=aga_RUL_percent_100_1dot5C.mat  SaveFormat=Timeseries
  To File1 : ToFile  Commented=on  Filename=RUL_percent_100_1dot5C.mat  SaveFormat=Timeseries
  To File2 : ToFile  Commented=on  Filename=SOC100  SaveFormat=Timeseries
  To File3 : ToFile  Commented=on  Filename=reg_temp2  SaveFormat=Timeseries
  To File4 : ToFile  Commented=on  Filename=conv_temp2  SaveFormat=Timeseries
  To File5 : ToFile  Commented=on  Filename=cycles80_2C2  SaveFormat=Timeseries
  To Workspace2 : ToWorkspace  Commented=on  VariableName=kWhr  SaveFormat=Timeseries  SampleTime=-1
  To Workspace4 : ToWorkspace  Commented=on  VariableName=SOC  SaveFormat=Timeseries  SampleTime=-1
  Voltage Sensor : fl_lib/Electrical/Electrical Sensors/Voltage Sensor
  base_adjustment : MATLAB Function  TreatAsAtomicUnit=on
  charge regulation1 : Subsystem
  cycle counter : Subsystem
  profile_iteration : Subsystem
  wires:
  PS-Simulink Converter/1 -> SOC Subsystem3/1(current), Scope/1  "current"
  PS-Simulink Converter1/1 -> Scope/2  "voltage"
  Subsystem/1(SOC) -> Scope1/1, Scope6/1  "og"
  PS-Simulink Converter5/1 -> To File3/1, Scope11/1
  Subsystem4/1(cycle) -> To File5/1, Display1/1, Scope29/1
  PS-Simulink Converter2/1 -> Scope10/1
  charge regulation1/1(y) -> Add2/1, Scope5/1
  profile_iteration/1(sig) -> Sum1/1, base_adjustment/1(sig), charge regulation1/2(sig)
  Sum1/1 -> Scope7/2, Gain2/1  "total"
  Signal Builder1/1(Signal 1) -> Gain5/1
  cycle counter/1(cnt) -> Subsystem4/1(y), Display/1
  profile_iteration/2(Out2) -> base_adjustment/2(t)
  base_adjustment/1(y) -> Sum1/2  "balancer"
  SOC Subsystem3/1(integrator) -> profile_iteration/1(subSOC), charge regulation1/1(subSOC), cycle counter/1(subSOC), Scope6/2, RUL Subsystem4/1(integrator)  "subSOC"
  Constant1/1 -> RUL Subsystem4/2(T)
  RUL Subsystem4/1(RUL) -> Scope12/1, To File1/1, To File/1
  PS-Simulink Converter3/1 -> Scope16/1
  Add2/1 -> Scope9/1, Simulink-PS Converter1/1
  Gain2/1 -> Add2/2, Gain4/1, Simulink-PS Converter/1, Scope7/1
  Gain4/1 -> Scope13/1
  Constant6/1 -> RUL Subsystem4/4(Cdch)
  connections:
  Subsystem/LConn1 -- Current Sensor/LConn1 -- Voltage Sensor/LConn1
  Controlled Current Source/LConn1 -- Current Sensor/RConn2
  Current Sensor/RConn1 -- PS-Simulink Converter/LConn1
  Voltage Sensor/RConn1 -- PS-Simulink Converter1/LConn1
  Simulink-PS Converter1/RConn1 -- Controlled Current Source/RConn1
  Temperature Sensor/LConn1 -- Subsystem11/LConn1
  Temperature Source/LConn1 -- Heat Flow Rate Sensor/RConn2
  PS-Simulink Converter5/LConn1 -- Temperature Sensor/RConn2
  Temperature Sensor/RConn1 -- Temperature Source1/LConn1
  PS-Simulink Converter2/LConn1 -- Heat Flow Rate Sensor/RConn1
  PS-Simulink Converter3/LConn1 -- Current Sensor1/RConn1
  Simulink-PS Converter/RConn1 -- Controlled Current Source1/RConn1
  Solver Configuration/RConn1 -- Subsystem/RConn1 -- Controlled Current Source/RConn2 -- Voltage Sensor/RConn2 -- Electrical Reference/LConn1

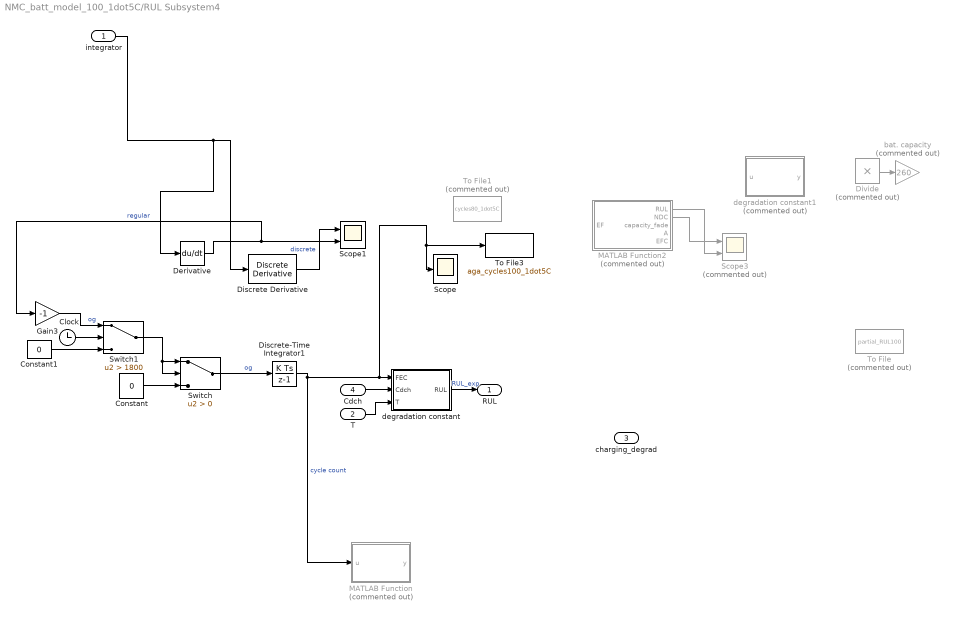
== system NMC_batt_model_100_1dot5C/RUL Subsystem4 ==
  integrator : Inport
  T : Inport  Port=2
  charging_degrad : Inport  Port=3
  Cdch : Inport  Port=4
  Clock : Clock
  Constant : Constant  Value=0
  Constant1 : Constant  Value=0
  Derivative : Derivative  CoefficientInTFapproximation=1000
  Discrete Derivative : simulink/Discrete/Discrete Derivative  gainval=1.0  ICPrevScaledInput=0.0  OutMin=[]  OutMax=[]  OutDataType=fixdt(1, 16)  OutScaling=2^-10  DoSatur=off
  Discrete-Time Integrator1 : DiscreteIntegrator  SampleTime=-1  ICPrevOutput=DiscIntNeverNeededParam  ICPrevScaledInput=DiscIntNeverNeededParam
  Divide : Product  Commented=on  Inputs=**
  Gain3 : Gain  Gain=-1
  MATLAB Function : MATLAB Function  Commented=on  TreatAsAtomicUnit=on
  MATLAB Function2 : MATLAB Function  Commented=on  TreatAsAtomicUnit=on
  Scope : Scope
  Scope1 : Scope  NumInputPorts=2
  Scope3 : Scope  Commented=on  NumInputPorts=2
  Switch : Switch  Criteria=u2 > Threshold  ZeroCross=off  SaturateOnIntegerOverflow=off  InputSameDT=off
  Switch1 : Switch  Criteria=u2 > Threshold  Threshold=1800  SaturateOnIntegerOverflow=off  InputSameDT=off
  To File : ToFile  Commented=on  Filename=partial_RUL100  SaveFormat=Timeseries
  To File1 : ToFile  Commented=on  Filename=cycles80_1dot5C  SaveFormat=Timeseries
  To File3 : ToFile  Filename=aga_cycles100_1dot5C
  bat. capacity : Gain  Commented=on  Gain=260
  degradation constant : MATLAB Function  TreatAsAtomicUnit=on
  degradation constant1 : MATLAB Function  Commented=on  TreatAsAtomicUnit=on
  RUL : Outport
  wires:
  Gain3/1 -> Switch1/1  "og"
  Constant/1 -> Switch/3
  Derivative/1 -> Gain3/1, Scope1/2  "regular"
  Discrete Derivative/1 -> Scope1/1  "discrete"
  Switch/1 -> Discrete-Time Integrator1/1  "og"
  integrator/1 -> Derivative/1, Discrete Derivative/1
  Discrete-Time Integrator1/1 -> MATLAB Function/1(u), To File3/1, Scope/1, degradation constant/1(FEC)  "cycle count"
  Clock/1 -> Switch1/2
  Constant1/1 -> Switch1/3
  Switch1/1 -> Switch/1, Switch/2
  Divide/1 -> bat. capacity/1
  MATLAB Function2/1(RUL) -> Scope3/2
  MATLAB Function2/2(NDC) -> Scope3/1
  Cdch/1 -> degradation constant/2(Cdch)
  T/1 -> degradation constant/3(T)
  degradation constant/1(RUL) -> RUL/1  "RUL_exp"

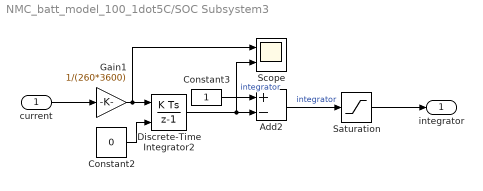
== system NMC_batt_model_100_1dot5C/SOC Subsystem3 ==
  current : Inport
  Add2 : Sum  Inputs=+-
  Constant2 : Constant  Value=0
  Constant3 : Constant
  Discrete-Time Integrator2 : DiscreteIntegrator  InitialConditionSource=external  SampleTime=-1  ICPrevOutput=DiscIntNeverNeededParam  ICPrevScaledInput=DiscIntNeverNeededParam
  Gain1 : Gain  Gain=1/(260*3600)
  Saturation : Saturate  UpperLimit=1  LowerLimit=0
  Scope : Scope  NumInputPorts=2
  integrator : Outport
  wires:
  Constant2/1 -> Discrete-Time Integrator2/2
  Constant3/1 -> Add2/1
  current/1 -> Gain1/1
  Gain1/1 -> Scope/1, Discrete-Time Integrator2/1
  Discrete-Time Integrator2/1 -> Scope/2, Add2/2  "integrator"
  Add2/1 -> Saturation/1  "integrator"
  Saturation/1 -> integrator/1
